simulink library "library_adpll"  (R2020a)
settings: Solver=ode45  StartTime=0.0  StopTime=10.0  RelTol=1e-3  EnableMultiTasking=on
values from neighbouring files (symbols this model uses):
  f0_dco = f0_dco0+gain_dco0*rand()    [pll_Nbit_vlsi_init.m]
  gain_dco = gain_dco0*(1+0.00*(rand-0.5))    [pll_Nbit_vlsi_init.m]
  integrator_init_state = Kint_den*(integrator_init_state_min+ 0.1*(integrator_init_state_max-integrator_init_state_min))    (= 419020.8)    [pll_Nbit_vlsi_init.m]
  Kint_den = 2^12    (= 4096)    [pll_Nbit_vlsi_init.m]
  Kint_num = 400    [pll_Nbit_vlsi_init.m]
  Kprop_den = 2^5    (= 32)    [pll_Nbit_vlsi_init.m]
  Kprop_num = 40    [pll_Nbit_vlsi_init.m]
  Nprop_in = 5    [pll_Nbit_vlsi_init.m]
  Nprop_out = 9    [pll_Nbit_vlsi_init.m]
  phi0 = rand*2*pi    [pll_Nbit_vlsi_init.m]
  tau = 30e-12    (= 3e-11)    [pll_Nbit_vlsi_init.m]
libraries: $bdroot x5, dspsigops x2
settings Model: Creator=galayko  LastModifiedBy=galayko
settings DataIOCC: LimitDataPoints=on  SaveFormat=Array  ReturnWorkspaceOutputs=off
settings OptimizationCC: LifeSpan=inf
settings DebuggingCC: SolverPrmCheckMsg=warning  SFUnexpectedBacktrackingDiag=warning  SFNoUnconditionalDefaultTransitionDiag=warning  ArithmeticOperatorsInVariantConditions=warning
settings HardwareCC: ProdBitPerPointer=32  ProdBitPerSizeT=32  ProdBitPerPtrDiffT=32  ProdLargestAtomicFloat=None  ProdIntDivRoundTo=Undefined  ProdEndianess=Unspecified  ProdWordSize=32  ProdHWDeviceType=32-bit Generic
settings ModelReferenceCC: PropagateSignalLabelsOutOfModel=off
settings SFSimCC: SimUseLocalCustomCode=off  CustomCodeUndefinedFunction=UseInterfaceOnly
settings RTWCC: RTWUseLocalCustomCode=off
settings CodeAppCC: StateflowObjectComments=on
settings GRTTargetCC: TargetLangStandard=C89/C90 (ANSI)
settings ConfigComp: CovMetricSettings=dw  CovHtmlReporting=on  CovSaveCumulativeToWorkspaceVar=on  CovSaveSingleToWorkspaceVar=on  CovExternalEMLEnable=off  CovSFcnEnable=off

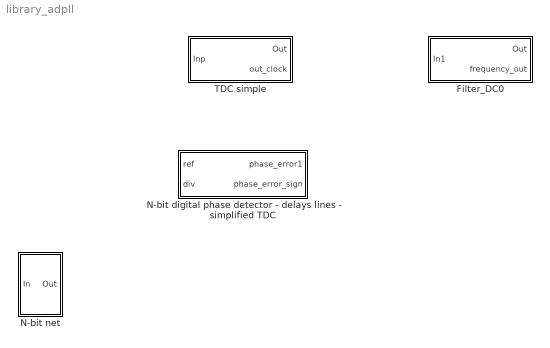
== system library_adpll ==
  Filter_DC0 : Subsystem  mask{Kprop_num=Kprop_num, Kprop_den=Kprop_den, Kint_num=Kint_num, Kint_den=Kint_den, f0_dco=f0_dco(1), gain_dco=gain_dco(1), phi0=phi0(1), integrator_init_state=integrator_init_state(1), Nprop_out=Nprop_out, Nprop_in=Nprop_in}
      mask prompts: Kprop_num "Proportional coef, numerator"; Kprop_den "Proportional coef, denominator"; Kint_num "Integral coef, numerator"; Kint_den "Integral coef, denominator"; f0_dco "DCO minimal frequency, Hz"; gain_dco "DCO frequency step, Hz"; phi0 "Initial phase, rad"; integrator_init_state "Initial state of accumulator"; Nprop_out "Number of bits of the proportional path output"; Nprop_in "Number of bits of the proportional path input"
      settings: MinAlgLoopOccurrences=on
  N-bit digital phase detector - delays lines - simplified TDC : Subsystem  TreatAsAtomicUnit=on  mask{T0=32e-12, D=0}
      mask prompts: T0 "Minimal delay"; D "Delay line parameter vector"
      settings: MinAlgLoopOccurrences=on
  N-bit net : Subsystem  TreatAsAtomicUnit=on  mask{n=0}
      mask prompts: n "Number of bit"
      settings: MinAlgLoopOccurrences=on
  TDC simple : Subsystem  TreatAsAtomicUnit=on  mask{tau=tau, max=14}
      mask prompts: tau "minimal delay"; max "maximal output"
      settings: MinAlgLoopOccurrences=on

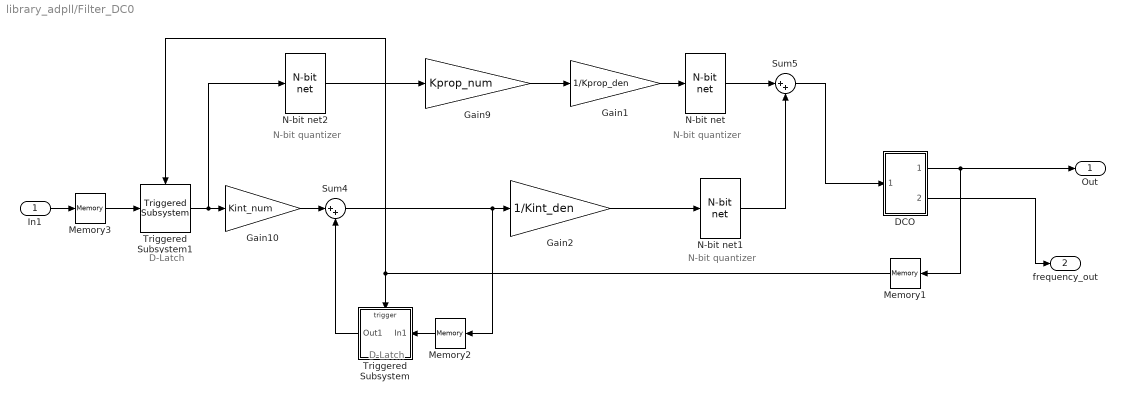
== system library_adpll/Filter_DC0 ==
  note: D-Latch
  note: N-bit quantizer
  note: N-bit quantizer
  note: N-bit quantizer
  note: D-Latch
  In1 : Inport
  DCO : Subsystem  TreatAsAtomicUnit=on  mask{f0=f0_dco, G=gain_dco, phi0=phi0}
      mask prompts: f0 "frequence centrale"; G "gain"; phi0 "Initial phase, rad"
      settings: MinAlgLoopOccurrences=on
  Gain1 : Gain  Gain=1/Kprop_den
  Gain10 : Gain  Gain=Kint_num
  Gain2 : Gain  Gain=1/Kint_den
  Gain9 : Gain  Gain=Kprop_num
  Memory1 : Memory
  Memory2 : Memory
  Memory3 : Memory
  N-bit net : $bdroot/N-bit net  n=Nprop_out
  N-bit net1 : $bdroot/N-bit net  n=11
  N-bit net2 : $bdroot/N-bit net  n=Nprop_in
  Sum4 : Sum  Inputs=|++
  Sum5 : Sum  Inputs=|++
  Triggered Subsystem : Subsystem  TreatAsAtomicUnit=on
  Triggered Subsystem1 : $bdroot/Filter_DC0/Triggered Subsystem  SystemSampleTime=-1  Latency=0  AutoFrameSizeCalculation=off
  Out : Outport
  frequency_out : Outport  Port=2
  wires:
  Memory1/1 -> Triggered Subsystem/Trigger, Triggered Subsystem1/Trigger
  N-bit net2/1 -> Gain9/1
  Triggered Subsystem1/1 -> N-bit net2/1, Gain10/1
  Memory3/1 -> Triggered Subsystem1/1
  Sum5/1 -> DCO/1(In1)
  N-bit net/1 -> Sum5/1
  Gain1/1 -> N-bit net/1
  N-bit net1/1 -> Sum5/2
  Triggered Subsystem/1(Out1) -> Sum4/2
  DCO/2(freq) -> frequency_out/1
  Gain2/1 -> N-bit net1/1
  Gain9/1 -> Gain1/1
  Gain10/1 -> Sum4/1
  Sum4/1 -> Memory2/1, Gain2/1
  In1/1 -> Memory3/1
  DCO/1(Out1) -> Memory1/1, Out/1
  Memory2/1 -> Triggered Subsystem/1(In1)

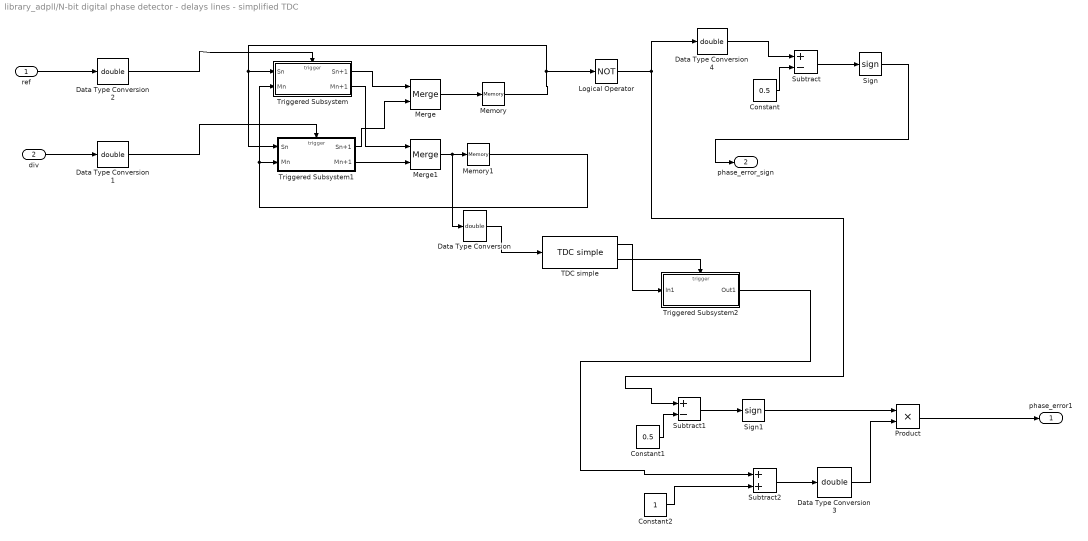
== system library_adpll/N-bit digital phase detector - delays lines - simplified TDC ==
  ref : Inport
  div : Inport  Port=2
  Constant : Constant  Value=0.5
  Constant1 : Constant  Value=0.5
  Constant2 : Constant
  Data Type Conversion{,1..4} (5 alike) : DataTypeConversion  OutDataTypeStr=double
  Logical Operator : Logic  Operator=NOT  AllPortsSameDT=off  OutDataTypeStr=boolean
  Memory : Memory
  Memory1 : Memory
  Merge : Merge
  Merge1 : Merge
  Product : Product  RndMeth=Zero
  Sign : Signum
  Sign1 : Signum
  Subtract : Sum  Inputs=+-
  Subtract1 : Sum  Inputs=+-
  Subtract2 : Sum
  TDC simple : $bdroot/TDC simple  tau=tau  max=14
  Triggered Subsystem : Subsystem  TreatAsAtomicUnit=on
  Triggered Subsystem1 : Subsystem  TreatAsAtomicUnit=on
  Triggered Subsystem2 : Subsystem  TreatAsAtomicUnit=on
      settings: MinAlgLoopOccurrences=on
  phase_error1 : Outport
  phase_error_sign : Outport  Port=2
  wires:
  Product/1 -> phase_error1/1
  TDC simple/1 -> Triggered Subsystem2/1(In1)
  Data Type Conversion3/1 -> Product/2
  Subtract2/1 -> Data Type Conversion3/1
  Sign1/1 -> Product/1
  Subtract1/1 -> Sign1/1
  Constant1/1 -> Subtract1/2
  Constant2/1 -> Subtract2/2
  Triggered Subsystem2/1(Out1) -> Subtract2/1
  Sign/1 -> phase_error_sign/1
  Data Type Conversion4/1 -> Subtract/1
  Subtract/1 -> Sign/1
  Constant/1 -> Subtract/2
  Logical Operator/1 -> Subtract1/1, Data Type Conversion4/1
  Memory1/1 -> Triggered Subsystem1/2(Mn), Triggered Subsystem/2(Mn)
  Data Type Conversion2/1 -> Triggered Subsystem/Trigger
  Data Type Conversion1/1 -> Triggered Subsystem1/Trigger
  Triggered Subsystem/1(Sn+1) -> Merge/1
  Triggered Subsystem/2(Mn+1) -> Merge1/1
  Triggered Subsystem1/1(Sn+1) -> Merge/2
  Triggered Subsystem1/2(Mn+1) -> Merge1/2
  Merge/1 -> Memory/1
  ref/1 -> Data Type Conversion2/1
  div/1 -> Data Type Conversion1/1
  Memory/1 -> Logical Operator/1, Triggered Subsystem/1(Sn), Triggered Subsystem1/1(Sn)
  Merge1/1 -> Memory1/1, Data Type Conversion/1
  Data Type Conversion/1 -> TDC simple/1
  TDC simple/2 -> Triggered Subsystem2/Trigger

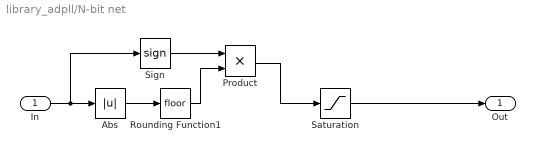
== system library_adpll/N-bit net ==
  In : Inport
  Abs : Abs
  Product : Product  RndMeth=Zero
  Rounding Function1 : Rounding
  Saturation : Saturate  UpperLimit=2^(n-1)-1  LowerLimit=-2^(n-1)
  Sign : Signum
  Out : Outport
  wires:
  Saturation/1 -> Out/1
  Product/1 -> Saturation/1
  Rounding Function1/1 -> Product/2
  Sign/1 -> Product/1
  Abs/1 -> Rounding Function1/1
  In/1 -> Sign/1, Abs/1

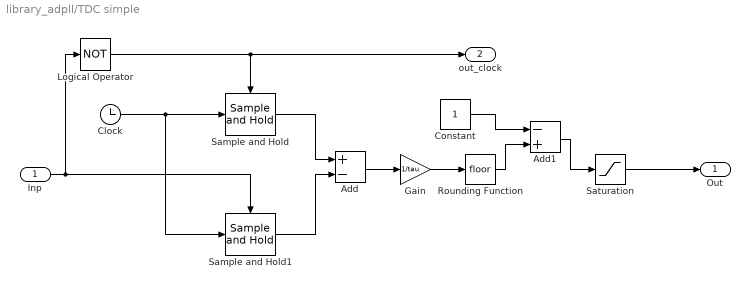
== system library_adpll/TDC simple ==
  Inp : Inport
  Add : Sum  Inputs=+-
  Add1 : Sum  Inputs=-+
  Clock : Clock
  Constant : Constant
  Gain : Gain  Gain=1/tau  OutMin=[0]
  Logical Operator : Logic  Operator=NOT  AllPortsSameDT=off  OutDataTypeStr=boolean
  Rounding Function : Rounding
  Sample and Hold : dspsigops/Sample and Hold  trig=Rising edge  initCond=0  latchinput=off
  Sample and Hold1 : dspsigops/Sample and Hold  trig=Rising edge  initCond=0  latchinput=off
  Saturation : Saturate  UpperLimit=max  LowerLimit=0
  Out : Outport
  out_clock : Outport  Port=2
  wires:
  Constant/1 -> Add1/1
  Rounding Function/1 -> Add1/2
  Add1/1 -> Saturation/1
  Clock/1 -> Sample and Hold/1, Sample and Hold1/1
  Inp/1 -> Sample and Hold1/Trigger, Logical Operator/1
  Sample and Hold/1 -> Add/1
  Sample and Hold1/1 -> Add/2
  Add/1 -> Gain/1
  Gain/1 -> Rounding Function/1
  Saturation/1 -> Out/1
  Logical Operator/1 -> out_clock/1, Sample and Hold/Trigger

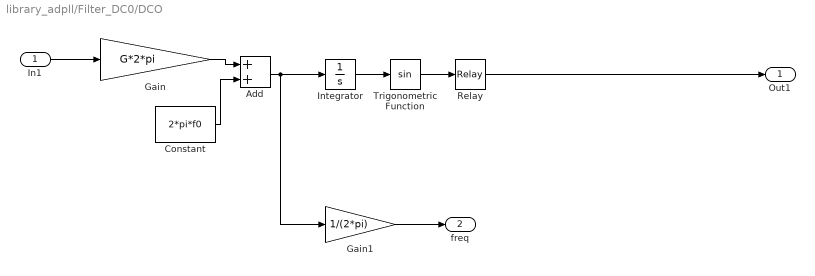
== system library_adpll/Filter_DC0/DCO ==
  In1 : Inport
  Add : Sum
  Constant : Constant  Value=2*pi*f0  SampleTime=0
  Gain : Gain  Gain=G*2*pi
  Gain1 : Gain  Gain=1/(2*pi)
  Integrator : Integrator  InitialCondition=phi0
  Relay : Relay  OnSwitchValue=0  OffSwitchValue=0  OffOutputValue=-1
  Trigonometric Function : Trigonometry
  Out1 : Outport
  freq : Outport  Port=2
  wires:
  Gain1/1 -> freq/1
  Relay/1 -> Out1/1
  In1/1 -> Gain/1
  Trigonometric Function/1 -> Relay/1
  Integrator/1 -> Trigonometric Function/1
  Add/1 -> Gain1/1, Integrator/1
  Gain/1 -> Add/1
  Constant/1 -> Add/2

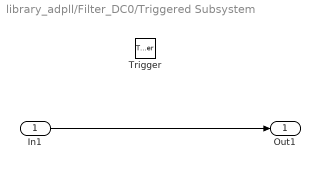
== system library_adpll/Filter_DC0/Triggered Subsystem ==
  In1 : Inport
  Trigger : TriggerPort  VariantControl=Variant
  Out1 : Outport
  wires:
  In1/1 -> Out1/1

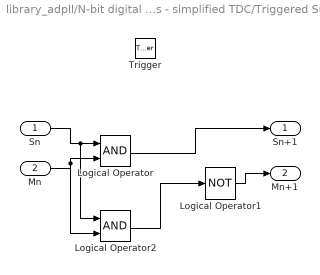
== system library_adpll/N-bit digital phase detector - delays lines - simplified TDC/Triggered Subsystem ==
  Sn : Inport
  Mn : Inport  Port=2
  Trigger : TriggerPort  VariantControl=Variant
  Logical Operator : Logic  AllPortsSameDT=off  OutDataTypeStr=boolean
  Logical Operator1 : Logic  Operator=NOT  AllPortsSameDT=off  OutDataTypeStr=boolean
  Logical Operator2 : Logic  AllPortsSameDT=off  OutDataTypeStr=boolean
  Sn+1 : Outport
  Mn+1 : Outport  Port=2
  wires:
  Sn/1 -> Logical Operator/1, Logical Operator2/1
  Mn/1 -> Logical Operator/2, Logical Operator2/2
  Logical Operator/1 -> Sn+1/1
  Logical Operator1/1 -> Mn+1/1
  Logical Operator2/1 -> Logical Operator1/1

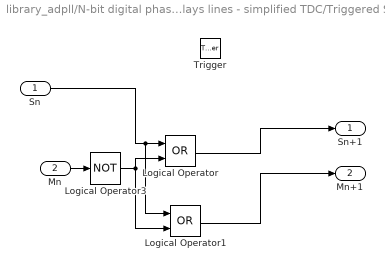
== system library_adpll/N-bit digital phase detector - delays lines - simplified TDC/Triggered Subsystem1 ==
  Sn : Inport
  Mn : Inport  Port=2
  Trigger : TriggerPort  VariantControl=Variant
  Logical Operator : Logic  Operator=OR  AllPortsSameDT=off  OutDataTypeStr=boolean
  Logical Operator1 : Logic  Operator=OR  AllPortsSameDT=off  OutDataTypeStr=boolean
  Logical Operator3 : Logic  Operator=NOT  AllPortsSameDT=off  OutDataTypeStr=boolean
  Sn+1 : Outport
  Mn+1 : Outport  Port=2
  wires:
  Sn/1 -> Logical Operator/1, Logical Operator1/1
  Mn/1 -> Logical Operator3/1
  Logical Operator/1 -> Sn+1/1
  Logical Operator1/1 -> Mn+1/1
  Logical Operator3/1 -> Logical Operator/2, Logical Operator1/2

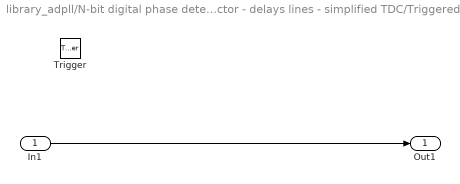
== system library_adpll/N-bit digital phase detector - delays lines - simplified TDC/Triggered Subsystem2 ==
  In1 : Inport
  Trigger : TriggerPort  VariantControl=Variant
  Out1 : Outport
  wires:
  In1/1 -> Out1/1
